simulink model "Accelerator_Observer"  (R2019a)
settings: Solver=FixedStepAuto  StartTime=0.0  StopTime=100000  RelTol=1e-3
settings Model: Creator=EiLit  LastModifiedBy=EiLit

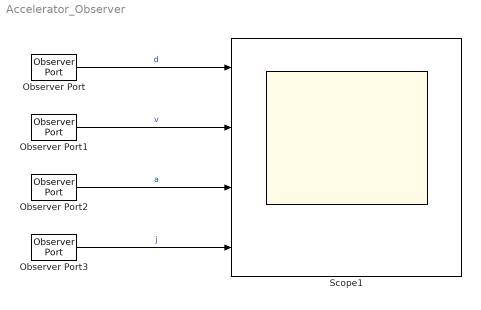
== system Accelerator_Observer ==
  Observer Port{,1..3} (4 alike) : ObserverPort
  Scope1 : Scope  NumInputPorts=4
  wires:
  Observer Port/1 -> Scope1/1  "d"
  Observer Port1/1 -> Scope1/2  "v"
  Observer Port2/1 -> Scope1/3  "a"
  Observer Port3/1 -> Scope1/4  "j"
